simulink model "AER821_LAB_1_S_V2"  (R2022b)
settings: Solver=ode113  StartTime=0.0  StopTime=T_sys  RelTol=1e-3
values from neighbouring files (symbols this model uses):
  d_Earth = -Pi_Luna * r_12    (= -4670658.19151)    [AER821_LAB_1.m]    (also in AER821_LAB_1_V2.m)
  d_Luna = Pi_Earth * r_12    (= 379729341.808)    [AER821_LAB_1.m]    (also in AER821_LAB_1_V2.m)
  Mu_Earth = G * M_Earth    (= 398716708000000)    [AER821_LAB_1.m]    (also in AER821_LAB_1_V2.m)
  Mu_Luna = G * M_Luna    (= 4904202160000)    [AER821_LAB_1.m]    (also in AER821_LAB_1_V2.m)
  Omega = sqrt(G * (M_Earth + M_Luna) / r_12^3)    [AER821_LAB_1.m]    (also in AER821_LAB_1_V2.m)
  r0x = xL1    [AER821_LAB_1.m]    (also in AER821_LAB_1_V2.m)
  r0y = 0    [AER821_LAB_1.m]    (also in AER821_LAB_1_V2.m)
  r0z = 0    [AER821_LAB_1.m]    (also in AER821_LAB_1_V2.m)
  v0x = 0    [AER821_LAB_1.m]    (also in AER821_LAB_1_V2.m)
  v0y = Omega * xL1    [AER821_LAB_1.m]    (also in AER821_LAB_1_V2.m)
  v0z = 0    [AER821_LAB_1.m]    (also in AER821_LAB_1_V2.m)
settings Model: Creator=Aidan  LastModifiedBy=Aidan

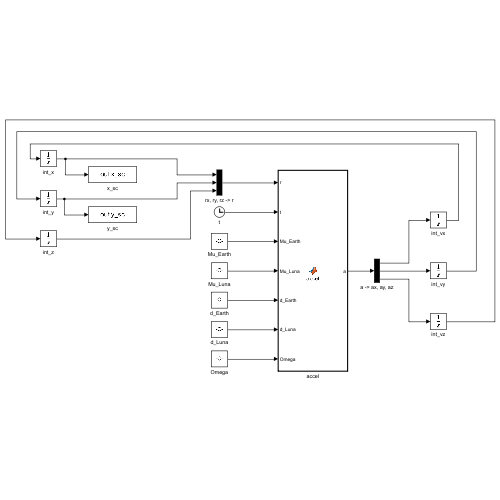
[thumbnail: Simulink's stored preview of the top-level diagram]
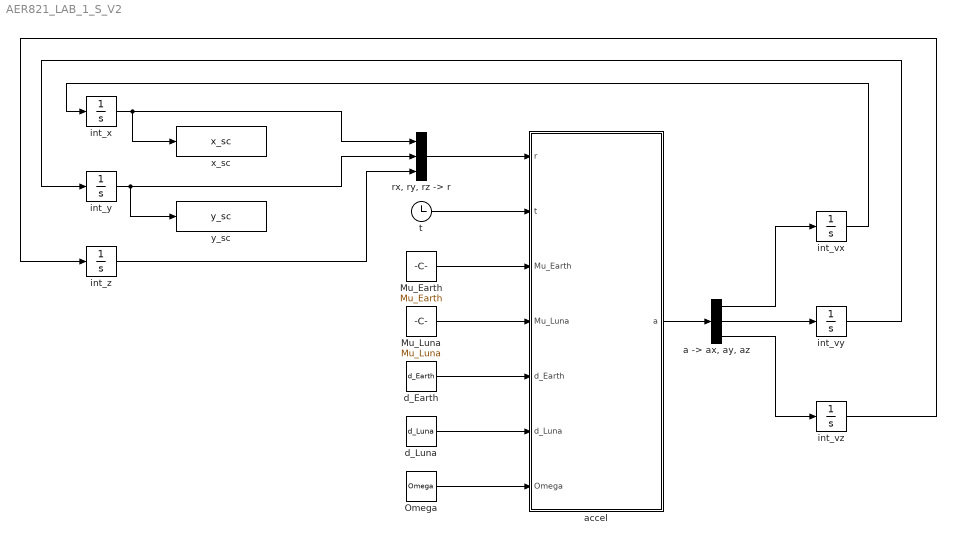
== system AER821_LAB_1_S_V2 ==
  Mu_Earth : Constant  Value=Mu_Earth
  Mu_Luna : Constant  Value=Mu_Luna
  Omega : Constant  Value=Omega
  "a -> ax, ay, az" : Demux  Outputs=3
  accel : MATLAB Function  TreatAsAtomicUnit=on
  d_Earth : Constant  Value=d_Earth
  d_Luna : Constant  Value=d_Luna
  int_vx : Integrator  InitialCondition=v0x
  int_vy : Integrator  InitialCondition=v0y
  int_vz : Integrator  InitialCondition=v0z
  int_x : Integrator  InitialCondition=r0x
  int_y : Integrator  InitialCondition=r0y
  int_z : Integrator  InitialCondition=r0z
  "rx, ry, rz -> r" : Mux  Inputs=3
  t : Clock
  x_sc : ToWorkspace  VariableName=x_sc  SaveFormat=Timeseries  SampleTime=-1
      settings: Save2DSignal=2-D array (concatenate along first dimension)
  y_sc : ToWorkspace  VariableName=y_sc  SaveFormat=Timeseries  SampleTime=-1
      settings: Save2DSignal=2-D array (concatenate along first dimension)
  wires:
  int_x/1 -> x_sc/1, "rx, ry, rz -> r"/1
  int_z/1 -> "rx, ry, rz -> r"/3
  "rx, ry, rz -> r"/1 -> accel/1(r)
  t/1 -> accel/2(t)
  d_Earth/1 -> accel/5(d_Earth)
  Omega/1 -> accel/7(Omega)
  d_Luna/1 -> accel/6(d_Luna)
  Mu_Luna/1 -> accel/4(Mu_Luna)
  Mu_Earth/1 -> accel/3(Mu_Earth)
  accel/1(a) -> "a -> ax, ay, az"/1
  "a -> ax, ay, az"/2 -> int_vy/1
  "a -> ax, ay, az"/1 -> int_vx/1
  "a -> ax, ay, az"/3 -> int_vz/1
  int_vx/1 -> int_x/1
  int_vy/1 -> int_y/1
  int_vz/1 -> int_z/1
  int_y/1 -> "rx, ry, rz -> r"/2, y_sc/1

== matlab function AER821_LAB_1_S_V2/accel ==
  data: r input; a output; t input; Mu_Earth input; Mu_Luna input; d_Earth input; d_Luna input; Omega input
function a = accel(r, t, Mu_Earth, Mu_Luna, d_Earth, d_Luna, Omega)

% Earth and Moon positions (barycenter frame)
RE = [d_Earth * cos(Omega * t); d_Earth * sin(Omega * t); 0];
RM = [d_Luna * cos(Omega * t);  d_Luna * sin(Omega * t); 0];

% Relative vectors
r1 = r - RE;
r2 = r - RM;

% Accelerations
a  = -Mu_Earth * r1 / (norm(r1)^3) -Mu_Luna  * r2 / (norm(r2)^3);
